simulink model "exercicio1lcsd2"  (R2026a)
settings: Solver=VariableStepAuto

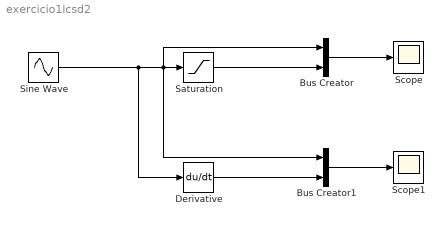
== system exercicio1lcsd2 ==
  Bus Creator : BusCreator  Inputs=2
  Bus Creator1 : BusCreator  Inputs=2
  Derivative : Derivative
  Saturation : Saturate
  Scope : Scope
  Scope1 : Scope
  Sine Wave : Sin  SampleTime=0
  wires:
  Saturation/1 -> Bus Creator/2
  Derivative/1 -> Bus Creator1/2
  Sine Wave/1 -> Derivative/1, Bus Creator/1, Bus Creator1/1, Saturation/1
  Bus Creator/1 -> Scope/1
  Bus Creator1/1 -> Scope1/1
